simulink model "2_2"  (R2018b)
settings: Solver=VariableStepAuto  StartTime=0.0  StopTime=30  RelTol=1e-3
libraries: fuzblock x1
settings Model: Creator=Konzem  LastModifiedBy=Konzem

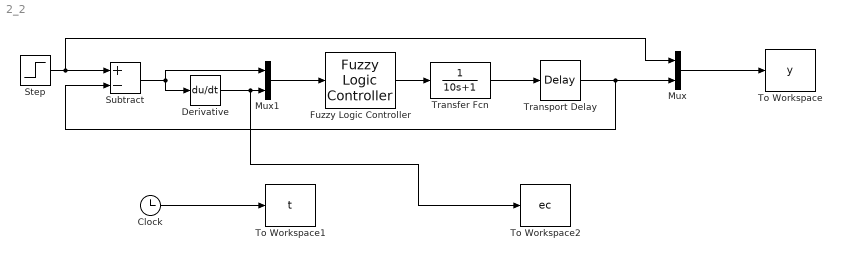
== system 2_2 ==
  Clock : Clock
  Derivative : Derivative
  Fuzzy Logic Controller : fuzblock/Fuzzy Logic  Controller  FIS=a2  OutputSampleNumber=101  DataType=double  FuzzifiedInputs=off  RuleFiringStrengths=off  RuleOutputs=off  AggregatedOutputs=off  SimulateUsing=Interpreted execution  OutOfRangeInputValueMessage=warning  NoRuleFiredMessage=warning  EmptyOutputFuzzySetMessage=warning
  Mux : Mux  Inputs=2
  Mux1 : Mux  Inputs=2
  Step : Step  Time=0  After=30  SampleTime=0
  Subtract : Sum  Inputs=+-
  To Workspace : ToWorkspace  VariableName=y  SampleTime=-1
      settings: Save2DSignal=2-D array (concatenate along first dimension)
  To Workspace1 : ToWorkspace  VariableName=t  SampleTime=-1
      settings: Save2DSignal=2-D array (concatenate along first dimension)
  To Workspace2 : ToWorkspace  VariableName=ec  SampleTime=-1
      settings: Save2DSignal=2-D array (concatenate along first dimension)
  Transfer Fcn : TransferFcn  Numerator=1  Denominator=[10 1]
  Transport Delay : TransportDelay  DelayTime=0.5
  wires:
  Clock/1 -> To Workspace1/1
  Transfer Fcn/1 -> Transport Delay/1
  Transport Delay/1 -> Subtract/2, Mux/2
  Fuzzy Logic Controller/1 -> Transfer Fcn/1
  Mux/1 -> To Workspace/1
  Step/1 -> Subtract/1, Mux/1
  Mux1/1 -> Fuzzy Logic Controller/1
  Subtract/1 -> Mux1/1, Derivative/1
  Derivative/1 -> To Workspace2/1, Mux1/2
